simulink model "LAB3"  (R2020a)
settings: Solver=VariableStepAuto  StartTime=0.0  StopTime=10.0  RelTol=1e-3
values from neighbouring files (symbols this model uses):
  beta = 1    [LAB_3.m]
  fm = La    (= 440)    [LAB_3.m]
libraries: commanabbnd3 x2
settings Model: Creator=danie  LastModifiedBy=danie

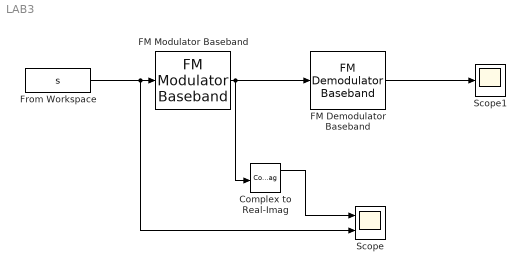
== system LAB3 ==
  Complex to Real-Imag : ComplexToRealImag
  "FM Demodulator Baseband " : commanabbnd3/FM Demodulator Baseband   FrequencyDeviation=75e3  SimulateUsing=Code generation
      settings: SourceProductBaseCode=CM
  FM Modulator Baseband : commanabbnd3/FM Modulator Baseband  FrequencyDeviation=beta*fm  SimulateUsing=Code generation
      settings: SourceProductBaseCode=CM
  From Workspace : FromWorkspace  VariableName=s
  Scope : Scope  NumInputPorts=2
  Scope1 : Scope
  wires:
  From Workspace/1 -> Scope/2, FM Modulator Baseband/1
  FM Modulator Baseband/1 -> "FM Demodulator Baseband "/1, Complex to Real-Imag/1
  Complex to Real-Imag/1 -> Scope/1
  "FM Demodulator Baseband "/1 -> Scope1/1
